simulink model "codebasedsimu"  (R2024b)
settings: Solver=ode4  StartTime=0.0  StopTime=5  FixedStep=0.005  RelTol=1e-3
values from neighbouring files (symbols this model uses):
  Ctrl_Trim = [0; -0.0964; 0; 0.6]    [Run_Validation.m]
  X0 = [ ... (first row only)    [Run_Validation.m]
settings Model: Creator=hw  LastModifiedBy=hw

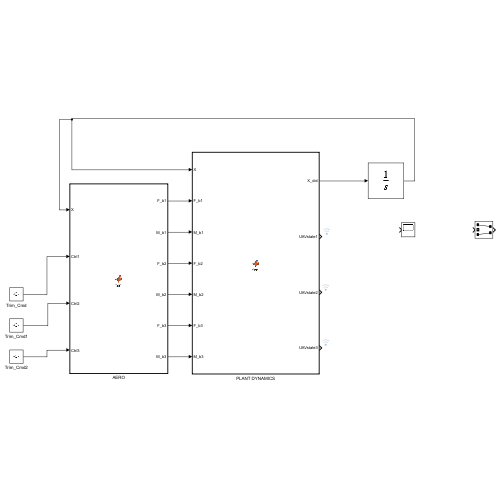
[thumbnail: Simulink's stored preview of the top-level diagram]
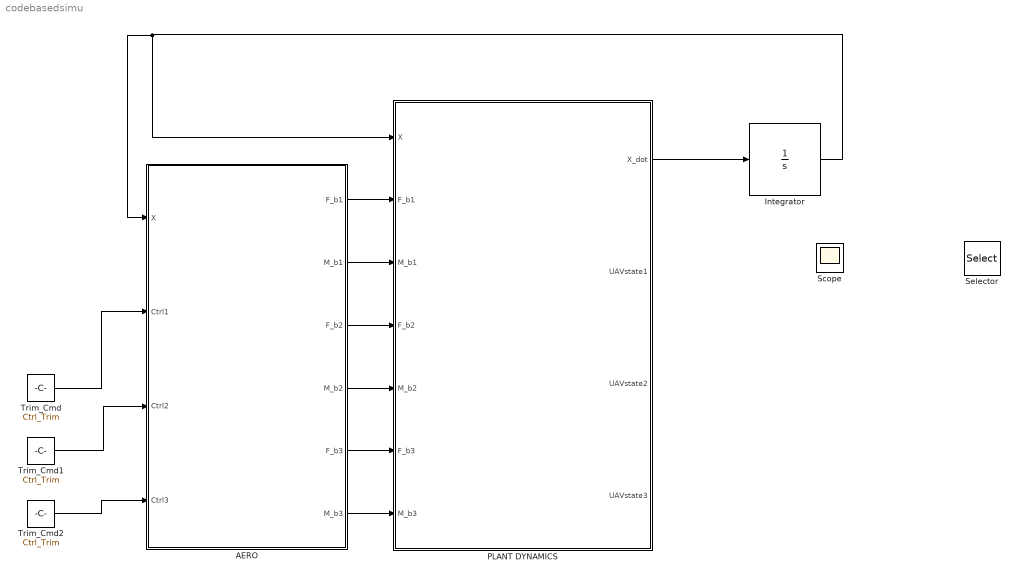
== system codebasedsimu ==
  AERO : MATLAB Function  TreatAsAtomicUnit=on
  Integrator : Integrator  InitialCondition=X0
  PLANT DYNAMICS : MATLAB Function  TreatAsAtomicUnit=on
  Scope : Scope
  Selector : Selector  InputPortWidth=3  IndexOptions=Index vector (dialog)  Indices=[1 3]  OutputSizes=1
  Trim_Cmd : Constant  Value=Ctrl_Trim
  Trim_Cmd1 : Constant  Value=Ctrl_Trim
  Trim_Cmd2 : Constant  Value=Ctrl_Trim
  wires:
  AERO/1(F_b1) -> PLANT DYNAMICS/2(F_b1)
  AERO/2(M_b1) -> PLANT DYNAMICS/3(M_b1)
  AERO/3(F_b2) -> PLANT DYNAMICS/4(F_b2)
  AERO/4(M_b2) -> PLANT DYNAMICS/5(M_b2)
  AERO/5(F_b3) -> PLANT DYNAMICS/6(F_b3)
  AERO/6(M_b3) -> PLANT DYNAMICS/7(M_b3)
  PLANT DYNAMICS/1(X_dot) -> Integrator/1
  Trim_Cmd/1 -> AERO/2(Ctrl1)
  Trim_Cmd1/1 -> AERO/3(Ctrl2)
  Trim_Cmd2/1 -> AERO/4(Ctrl3)
  Integrator/1 -> AERO/1(X), PLANT DYNAMICS/1(X)

== matlab function codebasedsimu/AERO ==
  data: X input; F_b1 output; Ctrl1 input; Ctrl2 input; Ctrl3 input; M_b1 output; F_b2 output; M_b2 output; F_b3 output; M_b3 output
function [F_b1, M_b1, F_b2, M_b2, F_b3, M_b3] = fcn(X, Ctrl1, Ctrl2, Ctrl3)
    [F_b1, M_b1, F_b2, M_b2, F_b3, M_b3] = ThreeBodyAerodynamics(X, Ctrl1, Ctrl2, Ctrl3)
end

== matlab function codebasedsimu/PLANT DYNAMICS ==
  data: X input; X_dot output; F_b1 input; M_b1 input; F_b2 input; M_b2 input; F_b3 input; M_b3 input; UAVstate1 output; UAVstate2 output; UAVstate3 output
function [X_dot, UAVstate1, UAVstate2, UAVstate3] = fcn(X, F_b1, M_b1, F_b2, M_b2, F_b3, M_b3)
    [X_dot, UAVstate1, UAVstate2, UAVstate3] = ThreeBodyDynamics(X, F_b1, M_b1, F_b2, M_b2, F_b3, M_b3);
end
